simulink library "util_frame_rotation_lib"  (R2015b)
settings: Solver=ode45  SolverMode=SingleTasking  StartTime=0.0  StopTime=10.0  RelTol=1e-3
values from neighbouring files (symbols this model uses):
  D = P*P*P + Q*Q    [mci2lla.m]
undefined symbols (not defined in the file or in its folder): central_body_omega_dot, de_cos_coeff, de_t_poly, e10coeff, e11coeff, e12coeff, e13coeff, e1coeff, e2coeff, e3coeff, e4coeff, e5coeff, e6coeff, e7coeff, e8coeff, e9coeff, earth_moon_rotation_matrix_select, ini_epoch_seconds, ini_hour, ini_minute, ini_moon_rotation_rate, ini_quat_mcmf_to_topo, ini_seconds, ini_tgt_landing_mcmf_pos, omega_moon_iau_coeff, omega_pa_mat_init, ra_sin_coeff, ra_t_poly
undefined symbols (not defined in the file): central_body_flattening, central_body_radius, central_body_rotation_rate
libraries: util_quat_lib x42, util_info_lib x21, util_common_lib x18, util_frame_rotation_lib x14, simulink_extras x9, util_extra_lib x4, simulink x2, util_orbit_dynamics_lib x1
(part 2 of 2)

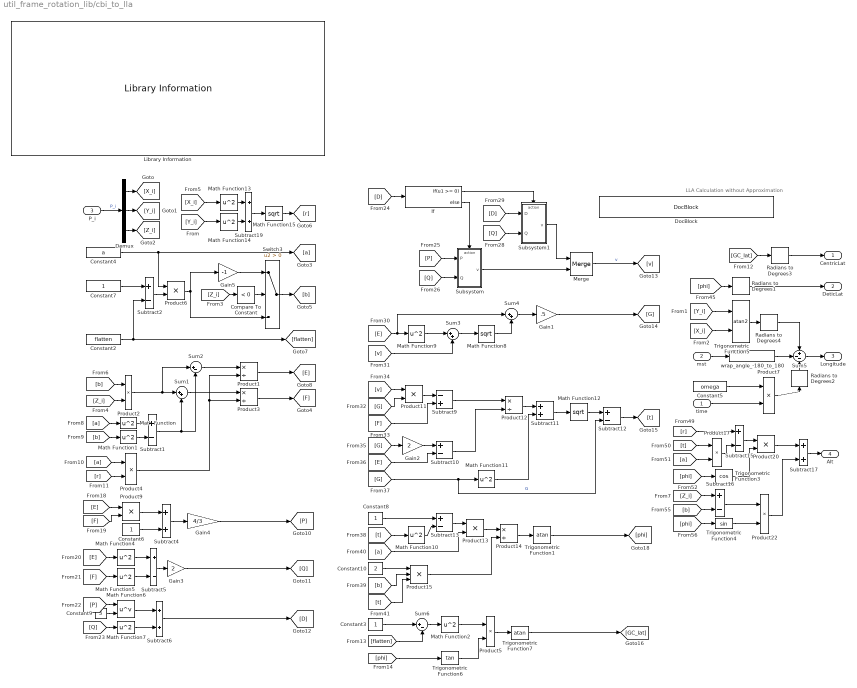
== system util_frame_rotation_lib/cbi_to_lla ==
  note: LLA Calculation without Approximation
  time : Inport
  mst : Inport  Port=2
  P_i : Inport  Port=3
  Compare To Constant : simulink/Logic and Bit Operations/Compare To Constant  relop=<  const=0  OutDataTypeStr=uint8
  Constant10 : Constant  Value=2
  Constant2 : Constant  Value=flatten
  Constant{3,6..8} (4 alike) : Constant
  Constant4 : Constant  Value=a
  Constant5 : Constant  Value=omega
  Constant9 : Constant  Value=3
  Demux : Demux  Outputs=3
  DocBlock : simulink/Model-Wide Utilities/DocBlock  DocumentType=Text
      content=|
      | function [latD, latC, lon, alt]  = cbi2lla( P_i, mst)
      | % FUNCTION cbi2lla
      | %   Compute Detic Latitude, Centric Latitude, Longitude, and Detic Altitude
      | %   from Central Body Inertial Coordinates
      | %
      | %   [latD, latC, lon, alt]  = cbi2lla( P_i, mst)
      | %
      | %  INPUTS
      | %   P_i         [1x3]   {m}         Position in Central Body Inertial Frame
      | %   mst         [1x1]   (degrees)   Mean Sidereal Time
      | %
      | %  OUTPUTS
      | %   detic_lat   [1x1]   {deg}       Detic Latitude
      | %   centric_lat [1x1]   {deg}       Centric Latitude
      | %   lon         [1x1]   {deg}       Longitude
      | %   alt         [1x1]   {m}         Detic Altitude
      | %
      | %  SOURCE
      | %   Borkowski, K.M. "Accurate Algorithms to Transform Geocentric to
      | %   Geodetic Coordinates"  Torun Radio Astronomy Observatory, Nicolaus
      | %   Copernicaus University, ul. Chopina 12/18, PL-87-100 Torun, Poland
      | %   Bullentin Geodesique, 63 (1989), pp. 50-56
      | %     http://www.astro.uni.torun.pl/~kb/Papers/geod/Geod-BG.htm
      |
      | %% Constants
      | R2D = 180.0/acos(-1);
      | D2R = acos(-1)/180.0;
      |
      | X = P_i(1);
      | Y = P_i(2);
      | Z = P_i(3);
      |
      | %% Compute Detic Latitude & Detic Altitude ==========================
      | r = sqrt( X*X + Y*Y );
      | if (Z < 0)
      |     b = -b;
      | end
      |
      | E = ((b*Z) - (a*a - b*b))/(a*r);        % {Eq 10}
      | F = ((b*Z) + (a*a - b*b))/(a*r);        % {Eq 11}
      |
      | P = (4/3)*(E*F + 1);                    % {Eq 16}
      | Q = 2*(E*E - F*F);                      % {Eq 17}
      |
      | D = (P*P*P) + (Q*Q);                    % {Eq 15}
      | if (D < 0)
      |     v = 2*(sqrt(-P))*cos( (1/2)*acos(Q/((-P)^(3/2))) );     % {Eq 14b}
      | else
      |     v = ((sqrt(D) - Q)^(1/3)) - ((sqrt(D) + Q)^(1/3));      % {Eq 14a}
      | end
      |
      | G = (sqrt(E*E + v) + E)/2;              % {Eq 13}
      | t = sqrt( G*G + (F-v*G)/(2*G-E)) - G;   % {Eq 12}
      |
      | phi = atan( a*(1-t*t)/(2*b*t) );        % {Eq 18}
      | h = (r-a*t)*cos(phi) + (Z-b)*sin(phi);  % {Eq 19}
      |
      | latD = phi * R2D;
      | alt = h;
      |
      | %% Compute Longitude ======================================================
      | lon = atan( Y / X ) * R2D - mst;
      |
      | %% Compute Centric Latitude ============================================
      | %   Centric Latitude {deg}
      | latC = atan((1 - flatten)^2 * tan(latD * D2R)) * R2D;
  Gain1 : Gain  Gain=.5
  Gain2 : Gain  Gain=2
  Gain3 : Gain  Gain=2
  Gain4 : Gain  Gain=4/3
  Gain5 : Gain  Gain=-1
  If : If  IfExpression=u1 >= 0
  Library Information : util_info_lib/Library Information  owner='NONE'
  Math Function{,1..2,4..5,7,9..11,13..14} (11 alike) : Math  Operator=square  SaturateOnIntegerOverflow=on
  Math Function12 : Math  Operator=sqrt  SaturateOnIntegerOverflow=on
  Math Function15 : Math  Operator=sqrt  SaturateOnIntegerOverflow=on
  Math Function6 : Math  Operator=pow  SaturateOnIntegerOverflow=on
  Math Function8 : Math  Operator=sqrt  SaturateOnIntegerOverflow=on
  Merge : Merge
  Product{1,3,12,14} (4 alike) : Product  Inputs=*/  RndMeth=Zero
  Product{5..6,11,13,17,20,22} (7 alike) : Product  Inputs=**  RndMeth=Zero
  Product15 : Product  Inputs=***  RndMeth=Zero
  Product2 : Product  RndMeth=Zero
  Product4 : Product  RndMeth=Zero
  Product7 : Product  Inputs=**  SaturateOnIntegerOverflow=on  OutDataTypeStr=Inherit: Same as first input
  Product9 : Product  RndMeth=Zero
  Radians to Degrees{1..4} (4 alike) : simulink_extras/Transformations/Radians to Degrees
  Subsystem : Subsystem
  Subsystem1 : Subsystem
  Subtract{1..2,5,10,12..13,15..16} (8 alike) : Sum  Inputs=+-
  Subtract{4,6,11,17,19} (5 alike) : Sum
  Subtract9 : Sum  Inputs=-+
  Sum1 : Sum  Inputs=|++
  Sum2 : Sum  Inputs=|+-
  Sum3 : Sum  Inputs=|++
  Sum4 : Sum  Inputs=|++
  Sum5 : Sum  Inputs=+--
  Sum6 : Sum  Inputs=|+-
  Switch3 : Switch  Criteria=u2 > Threshold
  Trigonometric Function1 : Trigonometry  Operator=atan
  Trigonometric Function3 : Trigonometry  Operator=cos
  Trigonometric Function4 : Trigonometry
  Trigonometric Function5 : Trigonometry  Operator=atan2
  Trigonometric Function6 : Trigonometry  Operator=tan
  Trigonometric Function7 : Trigonometry  Operator=atan
  wrap_angle_-180_to_180 : util_orbit_dynamics_lib/wrap_angle_-180_to_180  SystemSampleTime=-1
  CentricLat : Outport
  DeticLat : Outport  Port=2
  Longitude : Outport  Port=3
  Alt : Outport  Port=4
  wires:
  Gain5/1 -> Switch3/1
  Switch3/1 -> [b]
  Product6/1 -> Switch3/3, Gain5/1
  [Z_i] -> Compare To Constant/1
  Compare To Constant/1 -> Switch3/2
  Constant4/1 -> [a], Product6/1
  Constant7/1 -> Subtract2/1
  Constant2/1 -> [flatten], Subtract2/2
  Subtract2/1 -> Product6/2
  wrap_angle_-180_to_180/1 -> Sum5/2
  mst/1 -> wrap_angle_-180_to_180/1
  Radians to Degrees2/1 -> Sum5/3
  Constant5/1 -> Product7/1
  time/1 -> Product7/2
  Product7/1 -> Radians to Degrees2/1
  Sum5/1 -> Longitude/1
  Radians to Degrees4/1 -> Sum5/1
  Trigonometric Function5/1 -> Radians to Degrees4/1
  Radians to Degrees3/1 -> CentricLat/1
  Trigonometric Function7/1 -> [GC_lat]
  Product5/1 -> Trigonometric Function7/1
  Trigonometric Function6/1 -> Product5/2
  Math Function2/1 -> Product5/1
  [phi] -> Trigonometric Function6/1
  Sum6/1 -> Math Function2/1
  [flatten] -> Sum6/2
  Constant3/1 -> Sum6/1
  [GC_lat] -> Radians to Degrees3/1
  [Y_i] -> Trigonometric Function5/1
  [X_i] -> Trigonometric Function5/2
  Gain4/1 -> [P]
  Subtract1/1 -> Sum2/2, Sum1/2
  Sum2/1 -> Product1/1
  Product3/1 -> [F]
  Product1/1 -> [E]
  Math Function15/1 -> [r]
  Subtract19/1 -> Math Function15/1
  Math Function14/1 -> Subtract19/2
  Math Function13/1 -> Subtract19/1
  [Y_i] -> Math Function14/1
  [X_i] -> Math Function13/1
  Demux/3 -> [Z_i]
  Demux/2 -> [Y_i]
  Demux/1 -> [X_i]
  Subtract17/1 -> Alt/1
  Product22/1 -> Subtract17/2
  Product20/1 -> Subtract17/1
  Trigonometric Function4/1 -> Product22/2
  Subtract16/1 -> Product22/1
  [phi] -> Trigonometric Function4/1
  [Z_i] -> Subtract16/1
  [b] -> Subtract16/2
  Trigonometric Function3/1 -> Product20/2
  Subtract15/1 -> Product20/1
  [phi] -> Trigonometric Function3/1
  Radians to Degrees1/1 -> DeticLat/1
  Product17/1 -> Subtract15/2
  [r] -> Subtract15/1
  [a] -> Product17/2
  [t] -> Product17/1
  Trigonometric Function1/1 -> [phi]
  [phi] -> Radians to Degrees1/1
  Product14/1 -> Trigonometric Function1/1
  Product13/1 -> Product14/1
  Product15/1 -> Product14/2
  [t] -> Product15/3
  [b] -> Product15/2
  Constant10/1 -> Product15/1
  [a] -> Product13/2
  Subtract13/1 -> Product13/1
  Math Function10/1 -> Subtract13/2
  Constant8/1 -> Subtract13/1
  [t] -> Math Function10/1
  Subtract12/1 -> [t]
  Math Function12/1 -> Subtract12/1
  Subtract11/1 -> Math Function12/1
  Math Function11/1 -> Subtract11/2
  Product12/1 -> Subtract11/1
  [G] -> Subtract12/2, Math Function11/1  "G"
  Subtract10/1 -> Product12/2
  [E] -> Subtract10/2
  Gain2/1 -> Subtract10/1
  [G] -> Gain2/1
  Subtract9/1 -> Product12/1
  Product11/1 -> Subtract9/1
  [F] -> Subtract9/2
  [v] -> Product11/1
  [G] -> Product11/2
  Gain1/1 -> [G]
  Sum4/1 -> Gain1/1
  Math Function8/1 -> Sum4/2
  Sum3/1 -> Math Function8/1
  [v] -> Sum3/2
  Math Function9/1 -> Sum3/1
  [E] -> Sum4/1, Math Function9/1
  Merge/1 -> [v]  "v"
  Subsystem/1(v) -> Merge/2
  Subsystem1/1(v) -> Merge/1
  [D] -> Subsystem1/1(D)
  [Q] -> Subsystem1/2(Q)
  [Q] -> Subsystem/2(Q)
  [P] -> Subsystem/1(P)
  If/2 -> Subsystem/Action
  If/1 -> Subsystem1/Action
  [D] -> If/1
  Constant9/1 -> Math Function6/2
  Subtract6/1 -> [D]
  Math Function7/1 -> Subtract6/2
  Math Function6/1 -> Subtract6/1
  [Q] -> Math Function7/1
  [P] -> Math Function6/1
  Gain3/1 -> [Q]
  Subtract5/1 -> Gain3/1
  Math Function5/1 -> Subtract5/2
  Math Function4/1 -> Subtract5/1
  [F] -> Math Function5/1
  [E] -> Math Function4/1
  Subtract4/1 -> Gain4/1
  Product9/1 -> Subtract4/1
  Constant6/1 -> Subtract4/2
  [F] -> Product9/2
  [E] -> Product9/1
  Product4/1 -> Product1/2, Product3/2
  [r] -> Product4/2
  [a] -> Product4/1
  Sum1/1 -> Product3/1
  Math Function1/1 -> Subtract1/2
  Math Function/1 -> Subtract1/1
  [b] -> Math Function1/1
  [a] -> Math Function/1
  Product2/1 -> Sum2/1, Sum1/1
  [Z_i] -> Product2/2
  [b] -> Product2/1
  P_i/1 -> Demux/1  "P_i"

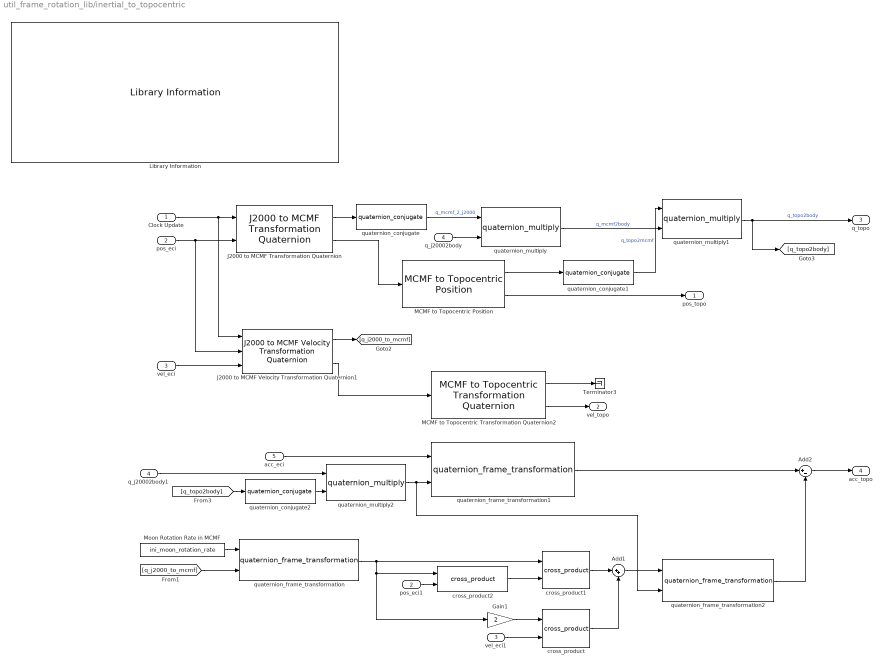
== system util_frame_rotation_lib/inertial_to_topocentric ==
  Clock Update : Inport
  pos_eci : Inport  Port=2
  vel_eci : Inport  Port=3
  q_j20002body : Inport  Port=4
  acc_eci : Inport  Port=5
  Add1 : Sum  Inputs=|++
  Add2 : Sum  Inputs=|+-
  Gain1 : Gain  Gain=2
  J2000 to MCMF Transformation Quaternion : util_frame_rotation_lib/J2000 to MCMF  Transformation Quaternion  SystemSampleTime=-1
  J2000 to MCMF Velocity Transformation Quaternion1 : util_frame_rotation_lib/J2000 to MCMF Velocity Transformation Quaternion  SystemSampleTime=-1
  Library Information : util_info_lib/Library Information  owner='NONE'
  MCMF to Topocentric Position : util_frame_rotation_lib/MCMF to Topocentric  Position  SystemSampleTime=-1
  MCMF to Topocentric Transformation Quaternion2 : util_frame_rotation_lib/MCMF to Topocentric  Transformation Quaternion  SystemSampleTime=-1
  Moon Rotation Rate in MCMF : Constant  Value=ini_moon_rotation_rate
  Terminator3 : Terminator
  cross_product : util_common_lib/cross_product  SystemSampleTime=-1
  cross_product1 : util_common_lib/cross_product  SystemSampleTime=-1
  cross_product2 : util_common_lib/cross_product  SystemSampleTime=-1
  pos_eci1 : InportShadow  Port=2
  q_j20002body1 : InportShadow  Port=4
  quaternion_conjugate : util_quat_lib/quaternion_conjugate  SystemSampleTime=-1
  quaternion_conjugate1 : util_quat_lib/quaternion_conjugate  SystemSampleTime=-1
  quaternion_conjugate2 : util_quat_lib/quaternion_conjugate  SystemSampleTime=-1
  quaternion_frame_transformation : util_quat_lib/quaternion_frame_transformation  SystemSampleTime=-1
  quaternion_frame_transformation1 : util_quat_lib/quaternion_frame_transformation  SystemSampleTime=-1
  quaternion_frame_transformation2 : util_quat_lib/quaternion_frame_transformation  SystemSampleTime=-1
  quaternion_multiply : util_quat_lib/quaternion_multiply  SystemSampleTime=-1
  quaternion_multiply1 : util_quat_lib/quaternion_multiply  SystemSampleTime=-1
  quaternion_multiply2 : util_quat_lib/quaternion_multiply  SystemSampleTime=-1
  vel_eci1 : InportShadow  Port=3
  pos_topo : Outport
  vel_topo : Outport  Port=2
  q_topo : Outport  Port=3
  acc_topo : Outport  Port=4
  wires:
  pos_eci/1 -> J2000 to MCMF Velocity Transformation Quaternion1/2, J2000 to MCMF Transformation Quaternion/2
  J2000 to MCMF Velocity Transformation Quaternion1/2 -> MCMF to Topocentric Transformation Quaternion2/1
  MCMF to Topocentric Position/2 -> pos_topo/1
  MCMF to Topocentric Transformation Quaternion2/1 -> Terminator3/1
  J2000 to MCMF Velocity Transformation Quaternion1/1 -> [q_j2000_to_mcmf]
  quaternion_multiply/1 -> quaternion_multiply1/2  "q_mcmf2body"
  quaternion_multiply1/1 -> [q_topo2body], q_topo/1  "q_topo2body"
  J2000 to MCMF Transformation Quaternion/1 -> quaternion_conjugate/1
  quaternion_conjugate/1 -> quaternion_multiply/1  "q_mcmf_2_j2000"
  q_j20002body/1 -> quaternion_multiply/2
  quaternion_conjugate1/1 -> quaternion_multiply1/1  "q_topo2mcmf"
  MCMF to Topocentric Position/1 -> quaternion_conjugate1/1
  MCMF to Topocentric Transformation Quaternion2/2 -> vel_topo/1
  vel_eci/1 -> J2000 to MCMF Velocity Transformation Quaternion1/3
  Clock Update/1 -> J2000 to MCMF Transformation Quaternion/1, J2000 to MCMF Velocity Transformation Quaternion1/1
  Add2/1 -> acc_topo/1
  q_j20002body1/1 -> quaternion_multiply2/1
  [q_topo2body] -> quaternion_conjugate2/1
  quaternion_conjugate2/1 -> quaternion_multiply2/2
  acc_eci/1 -> quaternion_frame_transformation1/1
  quaternion_frame_transformation1/1 -> Add2/1
  cross_product/1 -> Add1/2
  cross_product1/1 -> Add1/1
  pos_eci1/1 -> cross_product2/2
  cross_product2/1 -> cross_product1/2
  vel_eci1/1 -> cross_product/2
  Gain1/1 -> cross_product/1
  quaternion_frame_transformation/1 -> cross_product2/1, Gain1/1, cross_product1/1
  Moon Rotation Rate in MCMF/1 -> quaternion_frame_transformation/1
  [q_j2000_to_mcmf] -> quaternion_frame_transformation/2
  quaternion_multiply2/1 -> quaternion_frame_transformation1/2, quaternion_frame_transformation2/2
  quaternion_frame_transformation2/1 -> Add2/2
  Add1/1 -> quaternion_frame_transformation2/1
  J2000 to MCMF Transformation Quaternion/2 -> MCMF to Topocentric Position/1

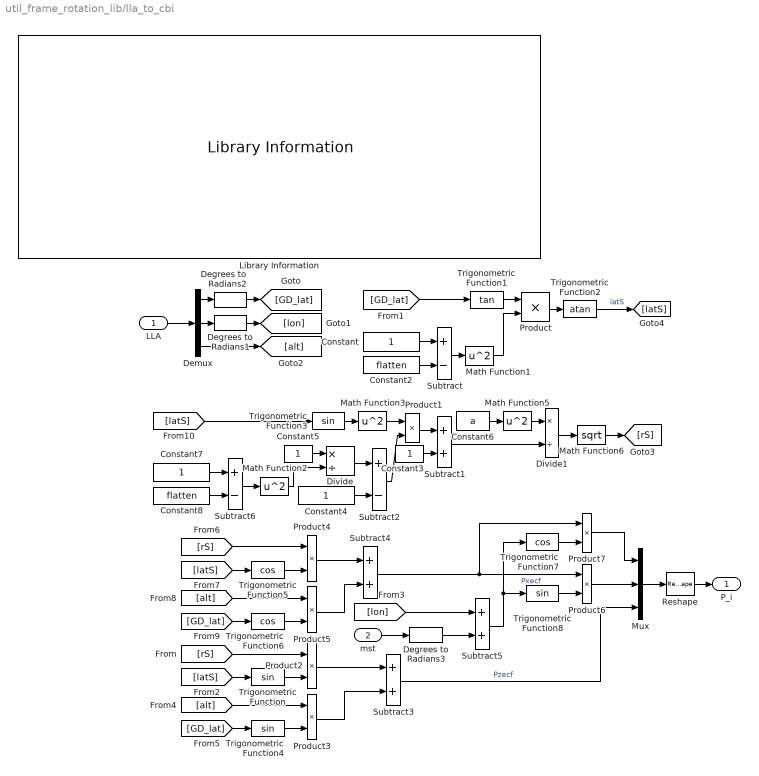
== system util_frame_rotation_lib/lla_to_cbi ==
  LLA : Inport
  mst : Inport  Port=2
  Constant{,3..5,7} (5 alike) : Constant
  Constant2 : Constant  Value=flatten
  Constant6 : Constant  Value=a
  Constant8 : Constant  Value=flatten
  Degrees to Radians1 : simulink_extras/Transformations/Degrees to Radians
  Degrees to Radians2 : simulink_extras/Transformations/Degrees to Radians
  Degrees to Radians3 : simulink_extras/Transformations/Degrees to Radians
  Demux : Demux  Outputs=3
  Divide : Product  Inputs=*/
  Divide1 : Product  Inputs=*/
  Library Information : util_info_lib/Library Information  owner='NONE'
  Math Function{1..3,5} (4 alike) : Math  Operator=square  SaturateOnIntegerOverflow=on
  Math Function6 : Math  Operator=sqrt  SaturateOnIntegerOverflow=on
  Mux : Mux  Inputs=3
  Product{,1..7} (8 alike) : Product  RndMeth=Zero
  Reshape : Reshape  OutputDimensionality=Column vector (2-D)
  Subtract : Sum  Inputs=+-
  Subtract{1,3..5} (4 alike) : Sum
  Subtract2 : Sum  Inputs=+-
  Subtract6 : Sum  Inputs=+-
  Trigonometric Function{,3..4,8} (4 alike) : Trigonometry
  Trigonometric Function1 : Trigonometry  Operator=tan
  Trigonometric Function2 : Trigonometry  Operator=atan
  Trigonometric Function5 : Trigonometry  Operator=cos
  Trigonometric Function6 : Trigonometry  Operator=cos
  Trigonometric Function7 : Trigonometry  Operator=cos
  P_i : Outport
  wires:
  Reshape/1 -> P_i/1
  LLA/1 -> Demux/1
  Demux/1 -> Degrees to Radians2/1
  Demux/2 -> Degrees to Radians1/1
  Demux/3 -> [alt]
  Degrees to Radians2/1 -> [GD_lat]
  Degrees to Radians1/1 -> [lon]
  Constant/1 -> Subtract/1
  Constant2/1 -> Subtract/2
  Subtract/1 -> Math Function1/1
  Math Function1/1 -> Product/2
  Constant3/1 -> Subtract1/2
  [GD_lat] -> Trigonometric Function1/1
  Trigonometric Function1/1 -> Product/1
  Product/1 -> Trigonometric Function2/1
  Trigonometric Function3/1 -> Math Function3/1
  Constant4/1 -> Subtract2/2
  Constant5/1 -> Divide/1
  Divide/1 -> Subtract2/1
  Subtract2/1 -> Product1/2
  Math Function3/1 -> Product1/1
  Product1/1 -> Subtract1/1
  Constant6/1 -> Math Function5/1
  Subtract1/1 -> Divide1/2
  Math Function5/1 -> Divide1/1
  Divide1/1 -> Math Function6/1
  Math Function6/1 -> [rS]
  [latS] -> Trigonometric Function/1
  Product2/1 -> Subtract3/1
  [GD_lat] -> Trigonometric Function4/1
  Product3/1 -> Subtract3/2
  [rS] -> Product2/1
  Trigonometric Function/1 -> Product2/2
  [alt] -> Product3/1
  Trigonometric Function4/1 -> Product3/2
  Subtract3/1 -> Mux/3  "Pzecf"
  Mux/1 -> Reshape/1
  [latS] -> Trigonometric Function5/1
  Product4/1 -> Subtract4/1
  [GD_lat] -> Trigonometric Function6/1
  Product5/1 -> Subtract4/2
  [rS] -> Product4/1
  Trigonometric Function5/1 -> Product4/2
  [alt] -> Product5/1
  Trigonometric Function6/1 -> Product5/2
  mst/1 -> Degrees to Radians3/1
  Degrees to Radians3/1 -> Subtract5/2
  [lon] -> Subtract5/1
  Subtract5/1 -> Trigonometric Function8/1, Trigonometric Function7/1
  Subtract4/1 -> Product6/1, Product7/1  "Pxecf"
  Trigonometric Function8/1 -> Product6/2
  Trigonometric Function7/1 -> Product7/2
  Product7/1 -> Mux/1
  Product6/1 -> Mux/2
  Trigonometric Function2/1 -> [latS]  "latS"
  [latS] -> Trigonometric Function3/1
  Constant7/1 -> Subtract6/1
  Constant8/1 -> Subtract6/2
  Subtract6/1 -> Math Function2/1
  Math Function2/1 -> Divide/2

== system util_frame_rotation_lib/q_eci_to_topo_DCM ==
  Clock Update : Inport
  q_J2000 : Inport  Port=2
  Ground : Ground
  J2000 to MCMF Transformation Quaternion : util_frame_rotation_lib/J2000 to MCMF  Transformation Quaternion  SystemSampleTime=-1
  Library Information : util_info_lib/Library Information  owner='NONE'
  MCMF to Topocentric Transformation Quaternion : util_frame_rotation_lib/MCMF to Topocentric  Transformation Quaternion  SystemSampleTime=-1
  Terminator1 : Terminator
  quaternion_conjugate : util_quat_lib/quaternion_conjugate  SystemSampleTime=-1
  quaternion_conjugate3 : util_quat_lib/quaternion_conjugate  SystemSampleTime=-1
  quaternion_conjugate4 : util_quat_lib/quaternion_conjugate  SystemSampleTime=-1
  quaternion_multiply : util_quat_lib/quaternion_multiply  SystemSampleTime=-1
  quaternion_multiply1 : util_quat_lib/quaternion_multiply  SystemSampleTime=-1
  quaternion_to_dcm : util_quat_lib/quaternion_to_dcm  SystemSampleTime=-1
  dcm : Outport
  wires:
  J2000 to MCMF Transformation Quaternion/2 -> MCMF to Topocentric Transformation Quaternion/1
  MCMF to Topocentric Transformation Quaternion/1 -> quaternion_conjugate3/1
  q_J2000/1 -> quaternion_multiply/2
  quaternion_conjugate4/1 -> quaternion_multiply/1
  J2000 to MCMF Transformation Quaternion/1 -> quaternion_conjugate4/1
  MCMF to Topocentric Transformation Quaternion/2 -> Terminator1/1
  Ground/1 -> J2000 to MCMF Transformation Quaternion/2
  Clock Update/1 -> J2000 to MCMF Transformation Quaternion/1
  quaternion_conjugate3/1 -> quaternion_multiply1/1
  quaternion_multiply/1 -> quaternion_multiply1/2
  quaternion_conjugate/1 -> quaternion_to_dcm/1
  quaternion_multiply1/1 -> quaternion_conjugate/1
  quaternion_to_dcm/1 -> dcm/1

== system util_frame_rotation_lib/quaternions_only ==
  Clock Update : Inport
  Add : Sum
  Divide : Product  Inputs=*/
  Library Information : util_info_lib/Library Information  owner='NONE'
  Moon Rotation Rate in MCMF : Constant  Value=ini_quat_mcmf_to_topo
  Moon and Earth EME2000 to Fixed Frame NEW : util_frame_rotation_lib/Moon and Earth  EME2000 to Fixed Frame NEW  SystemSampleTime=-1
  "Number of Days From Start of Julian Date to Jan 1, 2000 12:00:00" : Constant  Value=2451545
  Number of Seconds Per Day : Constant  Description=|  Value=86400
      | Number of Seconds                   
      | July 4, 2014 22:40:00 UTC           
      | Calculate on Web Site:              
      | www.mbari.org/staff/rich/utccalc.htm
  Terminator1 : Terminator
  Terminator5 : Terminator
  rotm_to_quaternion EME2000 to MCMF : util_extra_lib/rotm_to_quaternion
  q_J2000_to_MCMF : Outport
  q_MCMF_to_Topocentric : Outport  Port=2
  wires:
  Moon Rotation Rate in MCMF/1 -> q_MCMF_to_Topocentric/1
  Divide/1 -> Add/1
  Add/1 -> Moon and Earth EME2000 to Fixed Frame NEW/1
  Moon and Earth EME2000 to Fixed Frame NEW/3 -> Terminator1/1
  Moon and Earth EME2000 to Fixed Frame NEW/2 -> Terminator5/1
  "Number of Days From Start of Julian Date to Jan 1, 2000 12:00:00"/1 -> Add/2
  Clock Update/1 -> Divide/1  "Seconds Since Jan 1, 2000  12:00:00"
  rotm_to_quaternion EME2000 to MCMF/1 -> q_J2000_to_MCMF/1
  Number of Seconds Per Day/1 -> Divide/2
  Moon and Earth EME2000 to Fixed Frame NEW/1 -> rotm_to_quaternion EME2000 to MCMF/1

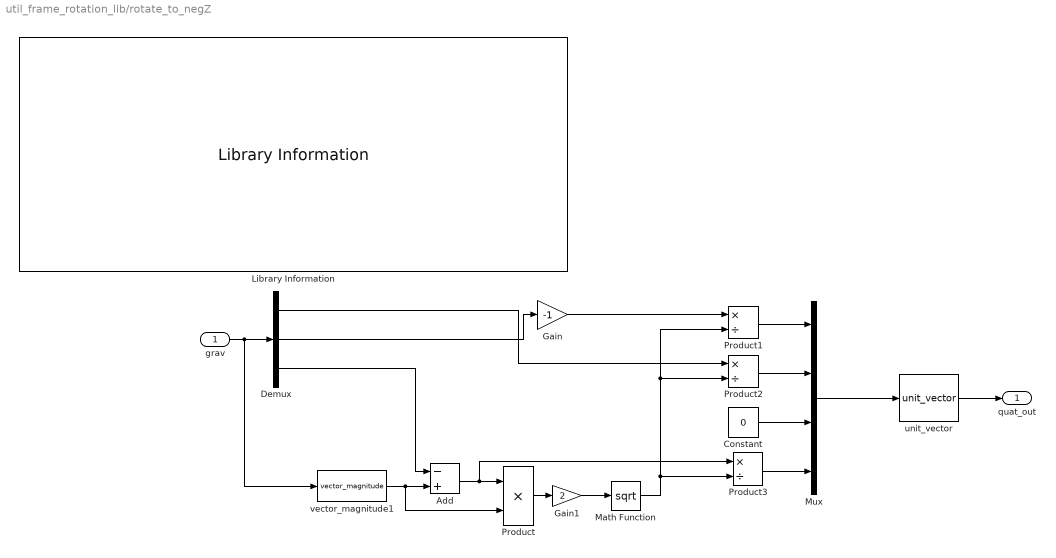
== system util_frame_rotation_lib/rotate_to_negZ ==
  grav : Inport
  Add : Sum  Inputs=-+
  Constant : Constant  Value=0
  Demux : Demux  Outputs=[1 1 1]
  Gain : Gain  Gain=-1
  Gain1 : Gain  Gain=2
  Library Information : util_info_lib/Library Information  owner='NONE'
  Math Function : Math  Operator=sqrt  SaturateOnIntegerOverflow=on
  Mux : Mux
  Product : Product  RndMeth=Zero
  Product1 : Product  Inputs=*/  RndMeth=Zero
  Product2 : Product  Inputs=*/  RndMeth=Zero
  Product3 : Product  Inputs=*/  RndMeth=Zero
  unit_vector : util_common_lib/unit_vector  SystemSampleTime=-1
  vector_magnitude1 : util_common_lib/vector_magnitude  SystemSampleTime=-1
  quat_out : Outport
  wires:
  Mux/1 -> unit_vector/1
  Product3/1 -> Mux/4
  Constant/1 -> Mux/3
  Demux/1 -> Product2/1
  Product2/1 -> Mux/2
  Product1/1 -> Mux/1
  Math Function/1 -> Product2/2, Product1/2, Product3/2
  Gain/1 -> Product1/1
  Demux/2 -> Gain/1
  Product/1 -> Gain1/1
  Add/1 -> Product3/1, Product/1
  Demux/3 -> Add/1
  vector_magnitude1/1 -> Product/2, Add/2
  grav/1 -> vector_magnitude1/1, Demux/1
  Gain1/1 -> Math Function/1
  unit_vector/1 -> quat_out/1

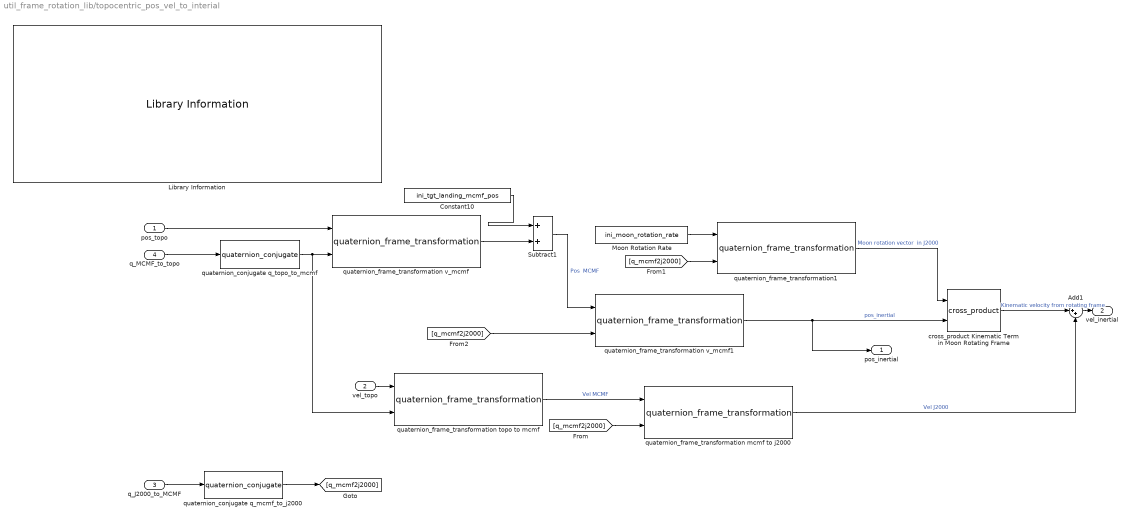
== system util_frame_rotation_lib/topocentric_pos_vel_to_interial ==
  pos_topo : Inport
  vel_topo : Inport  Port=2
  q_J2000_to_MCMF : Inport  Port=3
  q_MCMF_to_topo : Inport  Port=4
  Add1 : Sum  Inputs=|++
  Constant10 : Constant  Value=ini_tgt_landing_mcmf_pos
  Library Information : util_info_lib/Library Information  owner='NONE'
  Moon Rotation Rate : Constant  Value=ini_moon_rotation_rate
  Subtract1 : Sum
  cross_product Kinematic Term in Moon Rotating Frame : util_common_lib/cross_product  SystemSampleTime=-1
  quaternion_conjugate q_mcmf_to_j2000 : util_quat_lib/quaternion_conjugate  SystemSampleTime=-1
  quaternion_conjugate q_topo_to_mcmf : util_quat_lib/quaternion_conjugate  SystemSampleTime=-1
  quaternion_frame_transformation mcmf to j2000 : util_quat_lib/quaternion_frame_transformation  SystemSampleTime=-1
  quaternion_frame_transformation topo to mcmf : util_quat_lib/quaternion_frame_transformation  SystemSampleTime=-1
  quaternion_frame_transformation v_mcmf : util_quat_lib/quaternion_frame_transformation  SystemSampleTime=-1
  quaternion_frame_transformation v_mcmf1 : util_quat_lib/quaternion_frame_transformation  SystemSampleTime=-1
  quaternion_frame_transformation1 : util_quat_lib/quaternion_frame_transformation  SystemSampleTime=-1
  pos_inertial : Outport
  vel_inertial : Outport  Port=2
  wires:
  pos_topo/1 -> quaternion_frame_transformation v_mcmf/1
  q_MCMF_to_topo/1 -> quaternion_conjugate q_topo_to_mcmf/1
  quaternion_conjugate q_topo_to_mcmf/1 -> quaternion_frame_transformation topo to mcmf/2, quaternion_frame_transformation v_mcmf/2
  [q_mcmf2j2000] -> quaternion_frame_transformation1/2
  Subtract1/1 -> quaternion_frame_transformation v_mcmf1/1  "Pos  MCMF"
  vel_topo/1 -> quaternion_frame_transformation topo to mcmf/1
  quaternion_frame_transformation topo to mcmf/1 -> quaternion_frame_transformation mcmf to j2000/1  "Vel MCMF"
  Moon Rotation Rate/1 -> quaternion_frame_transformation1/1
  quaternion_frame_transformation1/1 -> cross_product Kinematic Term in Moon Rotating Frame/1  "Moon rotation vector  in J2000"
  Add1/1 -> vel_inertial/1
  quaternion_frame_transformation mcmf to j2000/1 -> Add1/2  "Vel J2000"
  cross_product Kinematic Term in Moon Rotating Frame/1 -> Add1/1  "Kinematic velocity from rotating frame"
  [q_mcmf2j2000] -> quaternion_frame_transformation mcmf to j2000/2
  q_J2000_to_MCMF/1 -> quaternion_conjugate q_mcmf_to_j2000/1
  quaternion_conjugate q_mcmf_to_j2000/1 -> [q_mcmf2j2000]
  [q_mcmf2j2000] -> quaternion_frame_transformation v_mcmf1/2
  quaternion_frame_transformation v_mcmf1/1 -> pos_inertial/1, cross_product Kinematic Term in Moon Rotating Frame/2  "pos_inertial"
  Constant10/1 -> Subtract1/1
  quaternion_frame_transformation v_mcmf/1 -> Subtract1/2

== system util_frame_rotation_lib/cbi_to_lla/Subsystem ==
  P : Inport
  Q : Inport  Port=2
  Action Port : ActionPort
  Constant9 : Constant  Value=3/2
  Gain1 : Gain  Gain=-1
  Gain3 : Gain  Gain=2
  Gain4 : Gain  Gain=1/2
  Math Function1 : Math  Operator=sqrt  SaturateOnIntegerOverflow=on
  Math Function6 : Math  Operator=pow  SaturateOnIntegerOverflow=on
  Product1 : Product  Inputs=*/  RndMeth=Zero
  Product6 : Product  Inputs=**  RndMeth=Zero
  Trigonometric Function : Trigonometry  Operator=cos
  Trigonometric Function1 : Trigonometry  Operator=acos
  v : Outport
  wires:
  Product6/1 -> v/1
  Trigonometric Function/1 -> Product6/2
  Gain4/1 -> Trigonometric Function/1
  Trigonometric Function1/1 -> Gain4/1
  Product1/1 -> Trigonometric Function1/1
  Math Function6/1 -> Product1/2
  Q/1 -> Product1/1  "Q"
  Constant9/1 -> Math Function6/2
  Gain3/1 -> Product6/1
  Math Function1/1 -> Gain3/1
  Gain1/1 -> Math Function6/1, Math Function1/1  "-P"
  P/1 -> Gain1/1

== system util_frame_rotation_lib/cbi_to_lla/Subsystem1 ==
  D : Inport
  Q : Inport  Port=2
  Action Port : ActionPort
  Constant2 : Constant  Value=1/3
  Constant3 : Constant  Value=1/3
  Math Function2 : Math  Operator=sqrt  SaturateOnIntegerOverflow=on
  Math Function3 : Math  Operator=pow  SaturateOnIntegerOverflow=on
  Math Function4 : Math  Operator=pow  SaturateOnIntegerOverflow=on
  Sum : Sum  Inputs=++|
  Sum1 : Sum  Inputs=|-+
  Sum2 : Sum  Inputs=+|-
  v : Outport
  wires:
  Sum2/1 -> v/1
  Math Function3/1 -> Sum2/1
  Math Function4/1 -> Sum2/2
  Sum1/1 -> Math Function3/1
  Constant3/1 -> Math Function3/2
  Q/1 -> Sum/2, Sum1/1  "Q"
  Sum/1 -> Math Function4/1
  Constant2/1 -> Math Function4/2
  Math Function2/1 -> Sum1/2, Sum/1
  D/1 -> Math Function2/1  "D"

== matlab function util_frame_rotation_lib/EML/EME2000 (J2000) to Moon Centered Moon Fixed (MCMF) ==
  data: xjdate input; tmatrix output; rasc_pole output; decl_pole output; moonrotationrate input
function [tmatrix, rasc_pole, decl_pole] = mm2000(xjdate,moonrotationrate)
%#codegen
% Version 0: 07292012 Jim Kaidy
% Compute Direction Cosine Matrix for International Astronomical Union
% (IAU)transformation from EME2000 (J2000) to model rotation of the Moon.
% xjdate == input current Terrestrial Barycenter Date (TDB) Julian Date and
% is defined as the number of days from start of Julian Calendar Jan 1,
% 4713 BC
% From "A Moon-Centered, Inertial Coordinate System for SPICE".


phat_moon = zeros(3,1);
xvec = zeros(1,3);
yvec = zeros(1,3);
zhat = zeros(3,1);
tmatrix = zeros(3);
omega_moon_pa_mat = zeros(3);
tmatrix_tod = zeros(3);

% Time Arguments

t = (xjdate - 2451545) / 36525;
d = xjdate - 2451545;

% IAU J2000 Pole Orientation

e1 = 125.045 -  0.0529921 * d; 
e2 = 250.089 -  0.1059842 * d; 
e3 = 260.008 + 13.0120009 * d; 
e4 = 176.625 + 13.3407154 * d; 
e5 = 357.529 +  0.9856003 * d; 
e6 = 311.589 + 26.4057084 * d; 
e7 = 134.963 + 13.0649930 * d; 
e8 = 276.617 +  0.3287146 * d; 
e9 =  34.226 +  1.7484877 * d;
e10 = 15.134 -  0.1589763 * d;
e11 =119.743 +  0.0036096 * d;
e12 =239.961 +  0.1643573 * d;
e13 = 25.053 + 12.9590088 * d; 
rasc_pole = 269.9949 + 0.0031 * t... 
           - 3.8787 * sind(e1)... 
           - 0.1204 * sind(e2)... 
           + 0.0700 * sind(e3)... 
           - 0.0172 * sind(e4)... 
           + 0.0072 * sind(e6)... 
           - 0.0052 * sind(e10)... 
           + 0.0043 * sind(e13); 
decl_pole = 66.5392 + 0.0130 * t... 
           + 1.5419 * cosd(e1)... 
           + 0.0239 * cosd(e2)... 
           - 0.0278 * cosd(e3)... 
           + 0.0068 * cosd(e4)... 
           - 0.0029 * cosd(e6)... 
           + 0.0009 * cosd(e7)... 
           + 0.0008 * cosd(e10)... 
           - 0.0009 * cosd(e13); 
       
% omega_dot_moon = 13.17635815; % moon rotation rate deg/day (1st order rate)
omega_dot_moon = 86400*(180/pi)*moonrotationrate(3);
if omega_dot_moon < 1
    omega_p = 0;
else
    omega_p = 38.3213 + omega_dot_moon * d - 1.4e-12 * d^2;
end

omega_moon_iau = omega_p + 3.5610 * sind(e1)...
                         + 0.1208 * sind(e2)...
                         - 0.0642 * sind(e3)...
                         + 0.0158 * sind(e4)...
                         + 0.0252 * sind(e5)...
                         - 0.0066 * sind(e6)...
                         - 0.0047 * sind(e7)...
                         - 0.0046 * sind(e8)...
                         + 0.0028 * sind(e9)...
                         + 0.0052 * sind(e10)...
                         + 0.0040 * sind(e11)...
                         + 0.0019 * sind(e12)...
                         - 0.0044 * sind(e13);
                     
rasc_moon_pa  = rasc_pole + 0.0553 * cosd(omega_p) + 0.0034 * cosd(omega_p + e1);
decl_moon_pa  = decl_pole + 0.0220 * sind(omega_p) + 0.0007 * sind(omega_p + e1);
omega_moon_pa = omega_moon_iau + 0.01775 - 0.0507 * cosd(omega_p) - 0.0034 * cosd(omega_p + e1);

omega_moon_pa_mat(1, 1) =  cosd(omega_moon_pa);
omega_moon_pa_mat(1, 2) =  sind(omega_moon_pa);
omega_moon_pa_mat(1, 3) =  0;
omega_moon_pa_mat(2, 1) =  -sind(omega_moon_pa);
omega_moon_pa_mat(2, 2) =  cosd(omega_moon_pa);
omega_moon_pa_mat(2, 3) =  0;
omega_moon_pa_mat(3, 1) =  0;
omega_moon_pa_mat(3, 2) =  0;
omega_moon_pa_mat(3, 3) =  1;

% Compute the unit vector in the direction of the moon's pole

phat_moon(1) = cosd(rasc_moon_pa) * cosd(decl_moon_pa); 
phat_moon(2) = sind(rasc_moon_pa) * cosd(decl_moon_pa); 
phat_moon(3) = sind(decl_moon_pa); 
phat_moon = phat_moon';

% Define EME2000 Z-Axis unit vector

zhat(1) = 0;
zhat(2) = 0;
zhat(3) = 1;

% Compute X-Axis unit vector

xvec = cross(zhat,phat_moon);
xhat = xvec/sqrt(xvec(1)^2 + xvec(2)^2 + xvec(3)^2);

% Compute Y-Axis direction

yvec = cross(phat_moon,xhat);
yhat = yvec/sqrt(yvec(1)^2 + yvec(2)^2 + yvec(3)^2);

% Load elements of transformation matrix

tmatrix_tod(1, 1) = xhat(1); 
tmatrix_tod(1, 2) = xhat(2); 
tmatrix_tod(1, 3) = xhat(3); 
tmatrix_tod(2, 1) = yhat(1); 
tmatrix_tod(2, 2) = yhat(2);
tmatrix_tod(2, 3) = yhat(3); 
tmatrix_tod(3, 1) = phat_moon(1); 
tmatrix_tod(3, 2) = phat_moon(2); 
tmatrix_tod(3, 3) = phat_moon(3);

tmatrix =  (tmatrix_tod'*omega_moon_pa_mat')';

end
